simulink library "NSA_DEVS_DIGITAL_LOGIC_COUPLED"  (R2023a)
settings: Solver=VariableStepAuto  StartTime=0.0  StopTime=10.0  RelTol=1e-3
libraries: $bdroot x22, NSA_DEVS_DIGITAL_LOGIC_ATOMIC x19
settings Model: Creator=david  LastModifiedBy=david

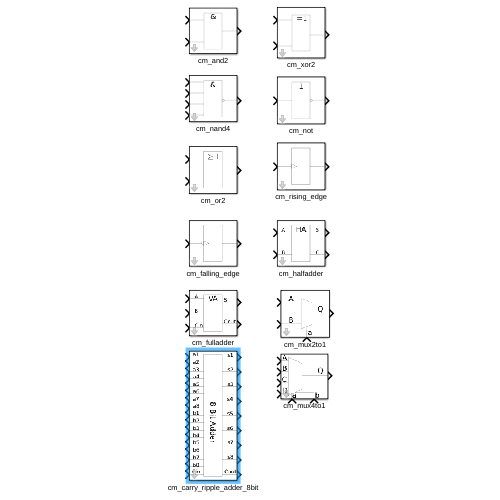
[thumbnail: Simulink's stored preview of the top-level diagram]
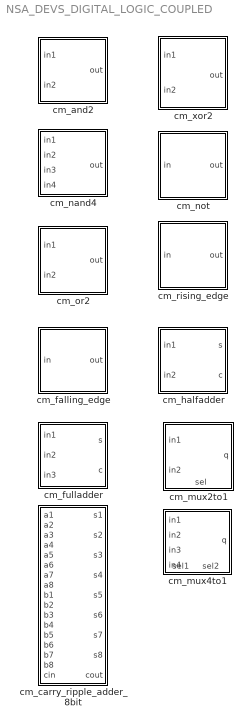
== system NSA_DEVS_DIGITAL_LOGIC_COUPLED ==
  cm_and2 : Subsystem  mask{tau=[0,1], debug=0}
  cm_carry_ripple_adder_8bit : Subsystem  mask{tau=[0,1], debug=0}
  cm_falling_edge : Subsystem  mask{tau=[0,1], debug=0}
  cm_fulladder : Subsystem  mask{tau=[0,1], debug=0}
  cm_halfadder : Subsystem  mask{tau=[0,1], debug=0}
  cm_mux2to1 : Subsystem  mask{tau=[0,1], debug=0}
      settings: PortSchema="{\"entries\":[{\"content\":{\"sides\":[{\"content\":{\"connectorIds\":[\"In1\",\"In2\"]},\"type\":\"ConnectorPlacement.EquallySpacedRectSide\",\"uuid\":\"34731d48-8e15-42ba-bd4b-aed28d23aea0\"},{\"content\":{\"connectorIds\":[\"Out1\"],\"side\":\"RIGHT\"},\"type\":\"ConnectorPlacement.EquallySpacedRectSide\",\"uuid\":\"a041c752-ab26-4ca5-92b4-ec2914ea875f\"},{\"content\":{\"side\":\"TOP\"},\"type\":\"ConnectorPlacement.EquallySpacedRectSide\",\"uuid\":\"d9c6c9da-164e-4da2-a825-82dcc4fc25b5\"},{\"content\":{\"connectorIds\":[\"In3\"],\"side\":\"BOTTOM\"},\"type\":\"ConnectorPlacement.EquallySpacedRectSide\",\"uuid\":\"cb6e077e-4478-4f88-a1c9-297156ed3aad\"}]},\"type\":\"ConnectorPlacement.EquallySpacedConnector\",\"uuid\":\"6a59c56d-0ca6-4e37-a002-1347e5691ec9\"}],\"packageUris\":[\"http://schema.mathworks.com/mf0/Connector/R2020b\"],\"version\":\"1.0\"}"
  cm_mux4to1 : Subsystem  mask{tau=[0,1], debug=0}
      settings: PortSchema="{\"entries\":[{\"content\":{\"sides\":[{\"content\":{\"connectorIds\":[\"In1\",\"In2\",\"In3\",\"In4\"]},\"type\":\"ConnectorPlacement.EquallySpacedRectSide\",\"uuid\":\"fc26a088-fa47-4166-98e4-908e63baa449\"},{\"content\":{\"connectorIds\":[\"Out1\"],\"side\":\"RIGHT\"},\"type\":\"ConnectorPlacement.EquallySpacedRectSide\",\"uuid\":\"3a4c553a-cbb7-43df-85ec-7cd09b4558b4\"},{\"content\":{\"side\":\"TOP\"},\"type\":\"ConnectorPlacement.EquallySpacedRectSide\",\"uuid\":\"55cc0d32-61c1-4296-9073-808d23534cef\"},{\"content\":{\"connectorIds\":[\"In5\",\"In6\"],\"side\":\"BOTTOM\"},\"type\":\"ConnectorPlacement.EquallySpacedRectSide\",\"uuid\":\"f37f76a1-a550-40f8-afa5-b24b9dbbb8a6\"}]},\"type\":\"ConnectorPlacement.EquallySpacedConnector\",\"uuid\":\"c29fc16c-eeff-4569-9d13-c6473d8cfb3a\"}],\"packageUris\":[\"http://schema.mathworks.com/mf0/Connector/R2020b\"],\"version\":\"1.0\"}"
  cm_nand4 : Subsystem  mask{tau=[0,1], debug=0}
  cm_not : Subsystem  mask{tau=[0,1], debug=0}
  cm_or2 : Subsystem  mask{tau=[0,1], debug=0}
  cm_rising_edge : Subsystem  mask{tau=[0,1], debug=0}
  cm_xor2 : Subsystem  mask{tau=[0,1], debug=0}

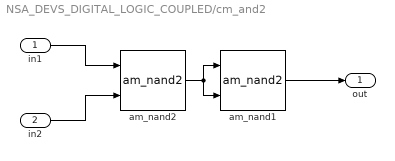
== system NSA_DEVS_DIGITAL_LOGIC_COUPLED/cm_and2 ==
  in1 : Inport
  in2 : Inport  Port=2
  am_nand1 : NSA_DEVS_DIGITAL_LOGIC_ATOMIC/am_nand2  tau=tau  debug=debug
      settings: SourceProductName=NSA_DEVS
  am_nand2 : NSA_DEVS_DIGITAL_LOGIC_ATOMIC/am_nand2  tau=tau  debug=debug
      settings: SourceProductName=NSA_DEVS
  out : Outport
  wires:
  in1/1 -> am_nand2/1
  in2/1 -> am_nand2/2
  am_nand2/1 -> am_nand1/2, am_nand1/1
  am_nand1/1 -> out/1

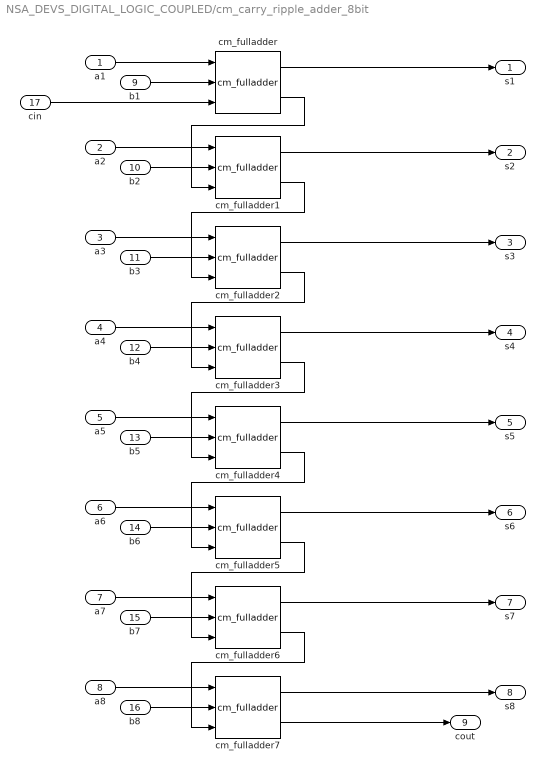
== system NSA_DEVS_DIGITAL_LOGIC_COUPLED/cm_carry_ripple_adder_8bit ==
  a1 : Inport
  a2 : Inport  Port=2
  a3 : Inport  Port=3
  a4 : Inport  Port=4
  a5 : Inport  Port=5
  a6 : Inport  Port=6
  a7 : Inport  Port=7
  a8 : Inport  Port=8
  b1 : Inport  Port=9
  b2 : Inport  Port=10
  b3 : Inport  Port=11
  b4 : Inport  Port=12
  b5 : Inport  Port=13
  b6 : Inport  Port=14
  b7 : Inport  Port=15
  b8 : Inport  Port=16
  cin : Inport  Port=17
  cm_fulladder{,1..7} (8 alike) : $bdroot/cm_fulladder  tau=tau  debug=debug
  s1 : Outport
  s2 : Outport  Port=2
  s3 : Outport  Port=3
  s4 : Outport  Port=4
  s5 : Outport  Port=5
  s6 : Outport  Port=6
  s7 : Outport  Port=7
  s8 : Outport  Port=8
  cout : Outport  Port=9
  wires:
  a1/1 -> cm_fulladder/1
  a2/1 -> cm_fulladder1/1
  a3/1 -> cm_fulladder2/1
  a4/1 -> cm_fulladder3/1
  a5/1 -> cm_fulladder4/1
  a6/1 -> cm_fulladder5/1
  a7/1 -> cm_fulladder6/1
  a8/1 -> cm_fulladder7/1
  b1/1 -> cm_fulladder/2
  b2/1 -> cm_fulladder1/2
  b3/1 -> cm_fulladder2/2
  b4/1 -> cm_fulladder3/2
  b5/1 -> cm_fulladder4/2
  b6/1 -> cm_fulladder5/2
  b7/1 -> cm_fulladder6/2
  b8/1 -> cm_fulladder7/2
  cm_fulladder/1 -> s1/1
  cm_fulladder1/1 -> s2/1
  cm_fulladder2/1 -> s3/1
  cm_fulladder3/1 -> s4/1
  cm_fulladder4/1 -> s5/1
  cm_fulladder5/1 -> s6/1
  cm_fulladder6/1 -> s7/1
  cm_fulladder7/1 -> s8/1
  cm_fulladder7/2 -> cout/1
  cin/1 -> cm_fulladder/3
  cm_fulladder/2 -> cm_fulladder1/3
  cm_fulladder1/2 -> cm_fulladder2/3
  cm_fulladder2/2 -> cm_fulladder3/3
  cm_fulladder3/2 -> cm_fulladder4/3
  cm_fulladder4/2 -> cm_fulladder5/3
  cm_fulladder5/2 -> cm_fulladder6/3
  cm_fulladder6/2 -> cm_fulladder7/3

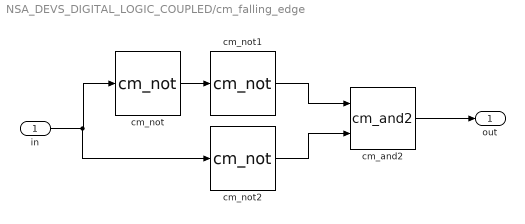
== system NSA_DEVS_DIGITAL_LOGIC_COUPLED/cm_falling_edge ==
  in : Inport
  cm_and2 : $bdroot/cm_and2  tau=tau  debug=debug
  cm_not : $bdroot/cm_not  tau=tau+[0,1]  debug=debug
  cm_not1 : $bdroot/cm_not  tau=tau+[0,1]  debug=debug
  cm_not2 : $bdroot/cm_not  tau=tau+[0,1]  debug=debug
  out : Outport
  wires:
  cm_not/1 -> cm_not1/1
  in/1 -> cm_not/1, cm_not2/1
  cm_not1/1 -> cm_and2/1
  cm_not2/1 -> cm_and2/2
  cm_and2/1 -> out/1

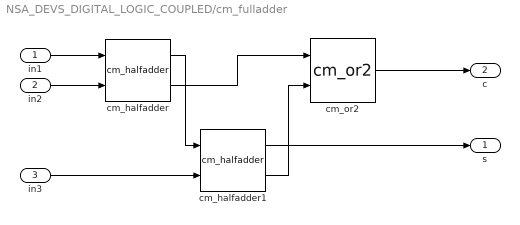
== system NSA_DEVS_DIGITAL_LOGIC_COUPLED/cm_fulladder ==
  in1 : Inport
  in2 : Inport  Port=2
  in3 : Inport  Port=3
  cm_halfadder : $bdroot/cm_halfadder  tau=tau  debug=debug
  cm_halfadder1 : $bdroot/cm_halfadder  tau=tau  debug=debug
  cm_or2 : $bdroot/cm_or2  tau=tau  debug=debug
  s : Outport
  c : Outport  Port=2
  wires:
  in1/1 -> cm_halfadder/1
  in2/1 -> cm_halfadder/2
  cm_halfadder/1 -> cm_halfadder1/1
  in3/1 -> cm_halfadder1/2
  cm_halfadder/2 -> cm_or2/1
  cm_halfadder1/2 -> cm_or2/2
  cm_halfadder1/1 -> s/1
  cm_or2/1 -> c/1

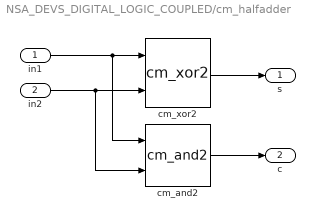
== system NSA_DEVS_DIGITAL_LOGIC_COUPLED/cm_halfadder ==
  in1 : Inport
  in2 : Inport  Port=2
  cm_and2 : $bdroot/cm_and2  tau=tau  debug=debug
  cm_xor2 : $bdroot/cm_xor2  tau=tau  debug=debug
  s : Outport
  c : Outport  Port=2
  wires:
  cm_xor2/1 -> s/1
  in1/1 -> cm_and2/1, cm_xor2/1
  in2/1 -> cm_and2/2, cm_xor2/2
  cm_and2/1 -> c/1

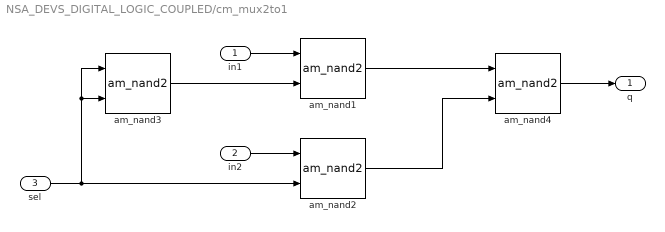
== system NSA_DEVS_DIGITAL_LOGIC_COUPLED/cm_mux2to1 ==
  in1 : Inport
  in2 : Inport  Port=2
  sel : Inport  Port=3
  am_nand{1..4} (4 alike) : NSA_DEVS_DIGITAL_LOGIC_ATOMIC/am_nand2  tau=tau  debug=debug
      settings: SourceProductName=NSA_DEVS
  q : Outport
  wires:
  in1/1 -> am_nand1/1
  in2/1 -> am_nand2/1
  sel/1 -> am_nand2/2, am_nand3/2, am_nand3/1
  am_nand3/1 -> am_nand1/2
  am_nand1/1 -> am_nand4/1
  am_nand2/1 -> am_nand4/2
  am_nand4/1 -> q/1

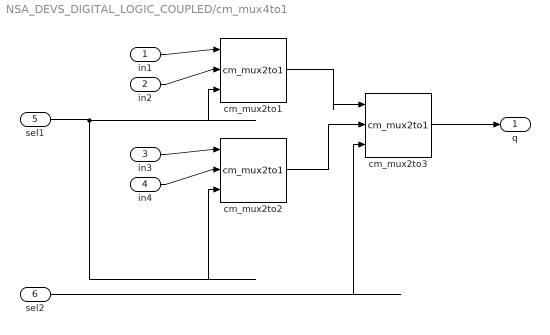
== system NSA_DEVS_DIGITAL_LOGIC_COUPLED/cm_mux4to1 ==
  in1 : Inport
  in2 : Inport  Port=2
  in3 : Inport  Port=3
  in4 : Inport  Port=4
  sel1 : Inport  Port=5
  sel2 : Inport  Port=6
  cm_mux2to1 : $bdroot/cm_mux2to1  tau=tau  debug=debug
  cm_mux2to2 : $bdroot/cm_mux2to1  tau=tau  debug=debug
  cm_mux2to3 : $bdroot/cm_mux2to1  tau=tau  debug=debug
  q : Outport
  wires:
  in1/1 -> cm_mux2to1/1
  in2/1 -> cm_mux2to1/2
  in4/1 -> cm_mux2to2/2
  in3/1 -> cm_mux2to2/1
  cm_mux2to1/1 -> cm_mux2to3/1
  cm_mux2to2/1 -> cm_mux2to3/2
  cm_mux2to3/1 -> q/1
  sel1/1 -> cm_mux2to2/3, cm_mux2to1/3
  sel2/1 -> cm_mux2to3/3

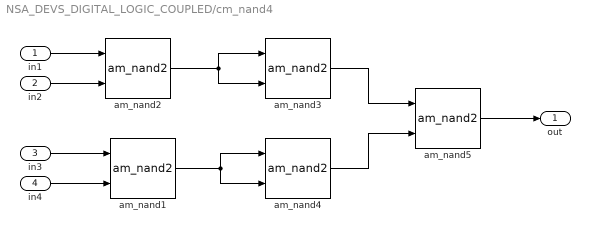
== system NSA_DEVS_DIGITAL_LOGIC_COUPLED/cm_nand4 ==
  in1 : Inport
  in2 : Inport  Port=2
  in3 : Inport  Port=3
  in4 : Inport  Port=4
  am_nand{1..5} (5 alike) : NSA_DEVS_DIGITAL_LOGIC_ATOMIC/am_nand2  tau=tau  debug=debug
      settings: SourceProductName=NSA_DEVS
  out : Outport
  wires:
  in1/1 -> am_nand2/1
  in2/1 -> am_nand2/2
  in3/1 -> am_nand1/1
  in4/1 -> am_nand1/2
  am_nand5/1 -> out/1
  am_nand2/1 -> am_nand3/2, am_nand3/1
  am_nand1/1 -> am_nand4/2, am_nand4/1
  am_nand4/1 -> am_nand5/2
  am_nand3/1 -> am_nand5/1

== system NSA_DEVS_DIGITAL_LOGIC_COUPLED/cm_not ==
  in : Inport
  am_nand2 : NSA_DEVS_DIGITAL_LOGIC_ATOMIC/am_nand2  tau=tau  debug=debug
      settings: SourceProductName=NSA_DEVS
  out : Outport
  wires:
  in/1 -> am_nand2/2, am_nand2/1
  am_nand2/1 -> out/1

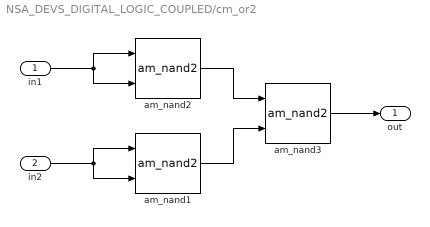
== system NSA_DEVS_DIGITAL_LOGIC_COUPLED/cm_or2 ==
  in1 : Inport
  in2 : Inport  Port=2
  am_nand1 : NSA_DEVS_DIGITAL_LOGIC_ATOMIC/am_nand2  tau=tau  debug=debug
      settings: SourceProductName=NSA_DEVS
  am_nand2 : NSA_DEVS_DIGITAL_LOGIC_ATOMIC/am_nand2  tau=tau  debug=debug
      settings: SourceProductName=NSA_DEVS
  am_nand3 : NSA_DEVS_DIGITAL_LOGIC_ATOMIC/am_nand2  tau=tau  debug=debug
      settings: SourceProductName=NSA_DEVS
  out : Outport
  wires:
  in1/1 -> am_nand2/2, am_nand2/1
  in2/1 -> am_nand1/1, am_nand1/2
  am_nand2/1 -> am_nand3/1
  am_nand1/1 -> am_nand3/2
  am_nand3/1 -> out/1

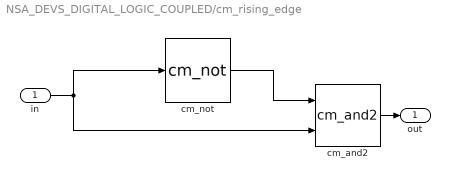
== system NSA_DEVS_DIGITAL_LOGIC_COUPLED/cm_rising_edge ==
  in : Inport
  cm_and2 : $bdroot/cm_and2  tau=tau  debug=debug
  cm_not : $bdroot/cm_not  tau=tau+[0,1]  debug=debug
  out : Outport
  wires:
  cm_and2/1 -> out/1
  in/1 -> cm_and2/2, cm_not/1
  cm_not/1 -> cm_and2/1

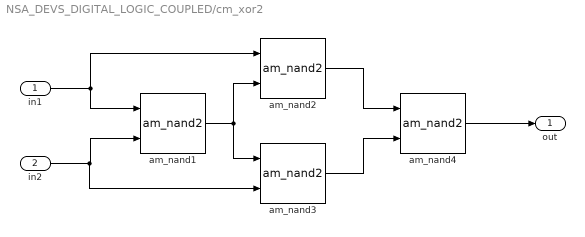
== system NSA_DEVS_DIGITAL_LOGIC_COUPLED/cm_xor2 ==
  in1 : Inport
  in2 : Inport  Port=2
  am_nand{1..4} (4 alike) : NSA_DEVS_DIGITAL_LOGIC_ATOMIC/am_nand2  tau=tau  debug=debug
      settings: SourceProductName=NSA_DEVS
  out : Outport
  wires:
  in1/1 -> am_nand2/1, am_nand1/1
  in2/1 -> am_nand3/2, am_nand1/2
  am_nand1/1 -> am_nand3/1, am_nand2/2
  am_nand2/1 -> am_nand4/1
  am_nand3/1 -> am_nand4/2
  am_nand4/1 -> out/1
